simulink model "ex08_1_1"  (R2023a)
settings: Solver=VariableStepAuto  StartTime=0.0  StopTime=15  MaxStep=1e-2  RelTol=1e-3
libraries: cstblocks x4, simulink x3
settings Model: Creator=sebe  LastModifiedBy=vigro
settings DebuggingCC: UnconnectedInputMsg=warning  UnconnectedOutputMsg=warning  UnconnectedLineMsg=warning
settings ModelReferenceCC: EnableRefExpFcnMdlSchedulingChecks=on
settings RTWCC: DLArmComputeVersion=19.05

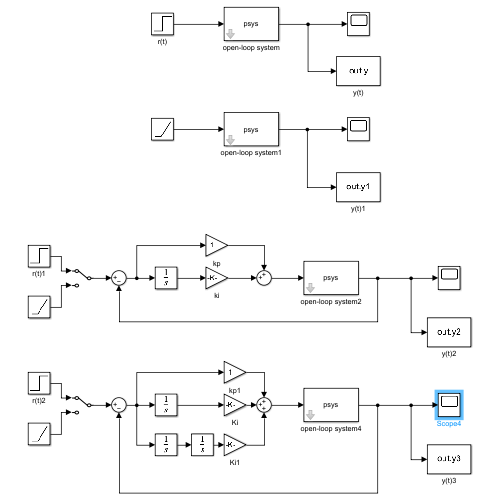
[thumbnail: Simulink's stored preview of the top-level diagram]
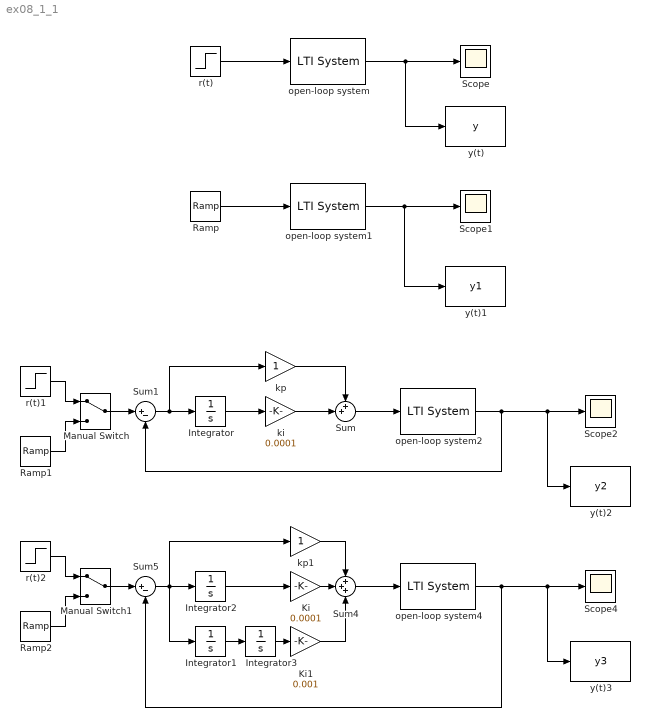
== system ex08_1_1 ==
  Integrator{,1..3} (4 alike) : Integrator
  Ki : Gain  Gain=0.0001
  Ki1 : Gain  Gain=0.001
  Manual Switch : ManualSwitch
  Manual Switch1 : ManualSwitch
  Ramp : simulink/Sources/Ramp  slope=1  start=0  InitialOutput=0
  Ramp1 : simulink/Sources/Ramp  slope=1  start=0  InitialOutput=0
  Ramp2 : simulink/Sources/Ramp  slope=1  start=0  InitialOutput=0
  Scope{,1..2,4} (4 alike) : Scope
  Sum : Sum  Inputs=++|
  Sum1 : Sum  Inputs=|+-
  Sum4 : Sum  Inputs=+++
  Sum5 : Sum  Inputs=|+-
  ki : Gain  Gain=0.0001
  kp : Gain
  kp1 : Gain
  open-loop system{,1..2,4} (4 alike) : cstblocks/LTI System  sys=psys  IC=[]
  r(t) : Step  Time=0  SampleTime=0
  r(t)1 : Step  Time=0  SampleTime=0
  r(t)2 : Step  Time=0  SampleTime=0
  y(t) : ToWorkspace  VariableName=y  SaveFormat=Timeseries  SampleTime=-1
  y(t)1 : ToWorkspace  VariableName=y1  SaveFormat=Timeseries  SampleTime=-1
  y(t)2 : ToWorkspace  VariableName=y2  SaveFormat=Timeseries  SampleTime=-1
  y(t)3 : ToWorkspace  VariableName=y3  SaveFormat=Timeseries  SampleTime=-1
  wires:
  r(t)/1 -> open-loop system/1
  open-loop system/1 -> Scope/1, y(t)/1
  Ramp/1 -> open-loop system1/1
  open-loop system1/1 -> y(t)1/1, Scope1/1
  Integrator/1 -> ki/1
  kp/1 -> Sum/1
  ki/1 -> Sum/2
  Sum/1 -> open-loop system2/1
  open-loop system2/1 -> y(t)2/1, Scope2/1, Sum1/2
  Sum1/1 -> kp/1, Integrator/1
  Sum5/1 -> Integrator1/1, kp1/1, Integrator2/1
  open-loop system4/1 -> y(t)3/1, Scope4/1, Sum5/2
  Sum4/1 -> open-loop system4/1
  kp1/1 -> Sum4/1
  Ki/1 -> Sum4/2
  Integrator2/1 -> Ki/1
  Manual Switch/1 -> Sum1/1
  r(t)1/1 -> Manual Switch/1
  Ramp1/1 -> Manual Switch/2
  Ramp2/1 -> Manual Switch1/2
  Manual Switch1/1 -> Sum5/1
  r(t)2/1 -> Manual Switch1/1
  Integrator1/1 -> Integrator3/1
  Integrator3/1 -> Ki1/1
  Ki1/1 -> Sum4/3
